simulink model "cuarto_de_auto"  (R2023b)
settings: Solver=VariableStepAuto  StartTime=0.0  StopTime=20  RelTol=1e-3
values from neighbouring files (symbols this model uses):
  A = [0 1 0 0;-k1/m1 -b1/m1 k1/m1 b1/m1;0 0 0 1;k2/m2 b1/m2 -(k1+k2)/m2 -b1/m2]    [cuarto_de_suspension_datos.m]
  B = [0 0;1/m1 0;0 0;-1/m2 k2/m2]    [cuarto_de_suspension_datos.m]
settings Model: Creator=Envy  LastModifiedBy=Envy

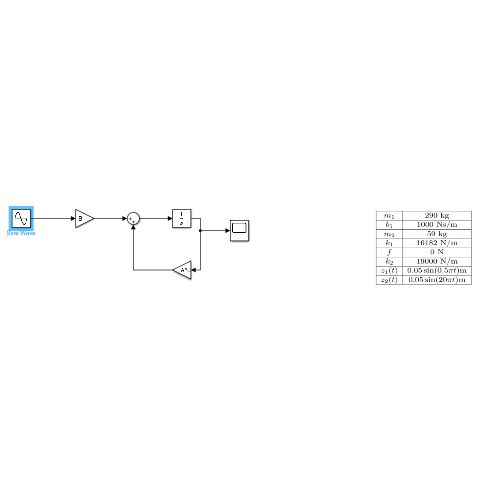
[thumbnail: Simulink's stored preview of the top-level diagram]
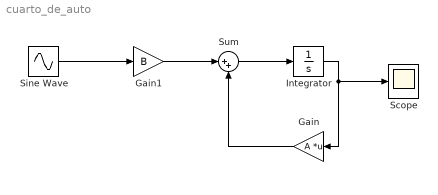
== system cuarto_de_auto ==
  Gain : Gain  Gain=A  Multiplication=Matrix(K*u)
  Gain1 : Gain  Gain=B
  Integrator : Integrator
  Scope : Scope
  Sine Wave : Sin  Amplitude=0.05  Frequency=0.5*pi  SampleTime=0
  Sum : Sum  Inputs=|++
  wires:
  Sum/1 -> Integrator/1
  Integrator/1 -> Gain/1, Scope/1
  Gain/1 -> Sum/2
  Gain1/1 -> Sum/1
  Sine Wave/1 -> Gain1/1
